simulink model "deliverable1_sim"  (R2025b)
settings: Solver=VariableStepAuto  StartTime=0.0  StopTime=110  RelTol=1e-3
settings Model: Creator=20212144  LastModifiedBy=20212144

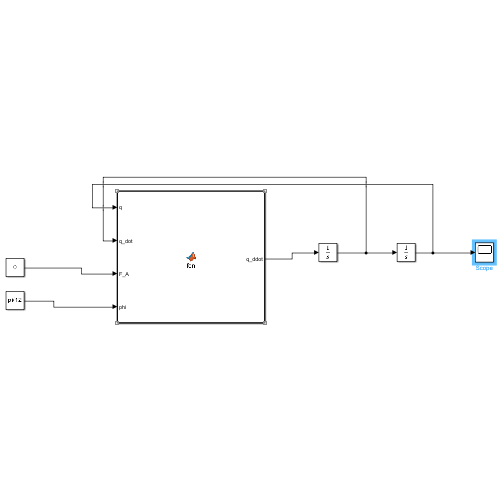
[thumbnail: Simulink's stored preview of the top-level diagram]
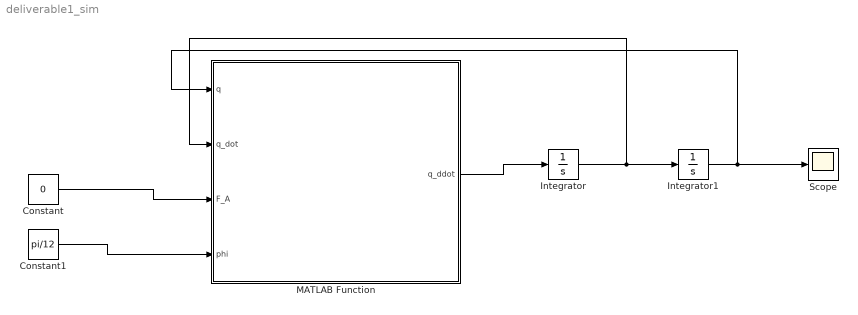
== system deliverable1_sim ==
  Constant : Constant  Value=0
  Constant1 : Constant  Value=pi/12
  Integrator : Integrator  InitialCondition=[0;0]
  Integrator1 : Integrator  InitialCondition=[11.5; 1/3*pi]
  MATLAB Function : MATLAB Function  TreatAsAtomicUnit=on
  Scope : Scope
      settings: ActiveDisplayYMinimum=-71.215477132524413  ActiveDisplayYMaximum=80.939093748845565
  wires:
  MATLAB Function/1(q_ddot) -> Integrator/1
  Integrator/1 -> MATLAB Function/2(q_dot), Integrator1/1
  Integrator1/1 -> Scope/1, MATLAB Function/1(q)
  Constant/1 -> MATLAB Function/3(F_A)
  Constant1/1 -> MATLAB Function/4(phi)

== matlab function deliverable1_sim/MATLAB Function ==
  data: q_ddot output; q input; q_dot input; F_A input; phi input
function q_ddot = fcn(q, q_dot, F_A, phi)

m_2 = 2e3;
m_3 = 500;
L_2 = 10; 
L_x = 12.5;
d_x = 200;
d_W = 2000;
k_theta = 200;
d_theta = 10;
k_x = 7000;
phi_dot = 0;
g=9.81;

theta = q(2);
theta_dot = q_dot(2);

x = q(1);
x_dot = q_dot(1);

M = [m_2 + m_3, -L_2*m_3*sin(phi - theta); -L_2*m_3*sin(phi - theta), L_2^2*m_3];
F = [F_A - d_x*x_dot + (m_3*(2*x*phi_dot^2 + cos(phi - theta)*phi_dot))/2 + (k_x*(2*L_x - 2*x))/2 + m_2*phi_dot^2*x - (g*m_2*sin(phi))/2 - g*m_3*sin(phi) - d_W*theta_dot*(sin(phi)*sin(theta) - cos(theta)^2) - L_2*m_3*theta_dot^2*cos(phi - theta) + L_2*m_3*phi_dot*theta_dot*cos(phi - theta); d_theta*(phi_dot - theta_dot) + (k_theta*(2*phi - 2*theta))/2 + L_2*g*m_3*cos(theta) + L_2*d_W*theta_dot*sin(2*theta) + (m_3*phi_dot*x*sin(phi - theta))/2 + L_2*m_3*phi_dot*x_dot*cos(phi - theta)];

q_ddot = M \ F;
end
